simulink model "pid_controller"  (R2021b)
settings: Solver=VariableStepAuto  StartTime=0.0  StopTime=10.0  RelTol=1e-3
values from neighbouring files (symbols this model uses):
  Kd = 0.5    [init.m]
  Ki = 1    [init.m]
  Kp = 0.001    [init.m]    (also in init.mat = 1)
settings Model: Creator=lordx  LastModifiedBy=lordx

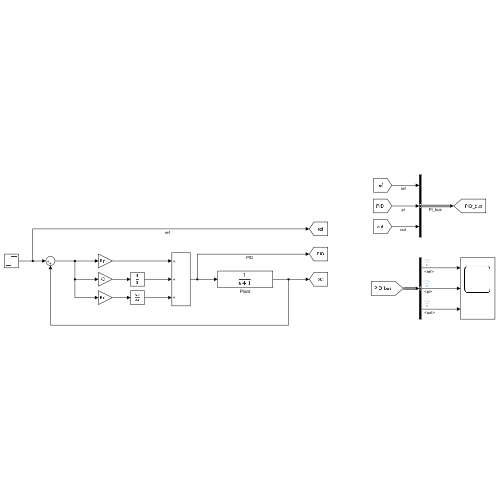
[thumbnail: Simulink's stored preview of the top-level diagram]
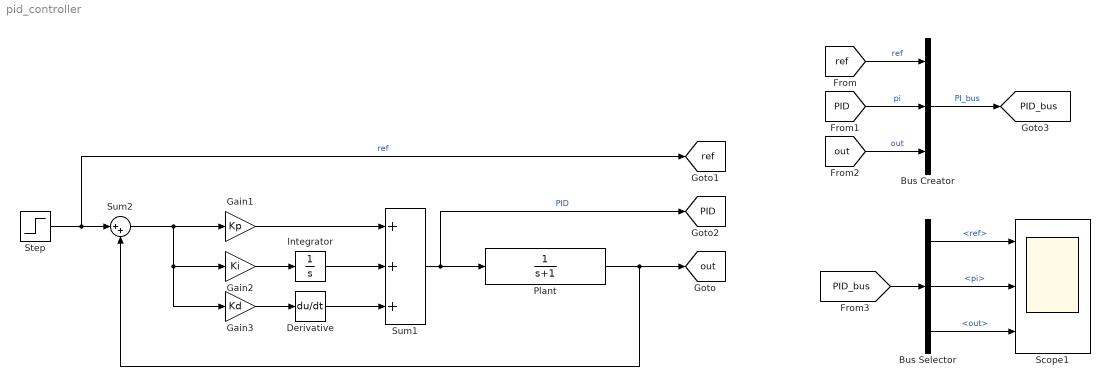
== system pid_controller ==
  Bus Selector : BusSelector  OutputSignals=ref,pi,out
  Bus Creator : BusCreator  Inputs=3
  Derivative : Derivative
  Gain1 : Gain  Gain=Kp
  Gain2 : Gain  Gain=Ki
  Gain3 : Gain  Gain=Kd
  Integrator : Integrator
  Plant : TransferFcn  Denominator=[1 1]
  Scope1 : Scope  NumInputPorts=3
  Step : Step  Time=0  SampleTime=0
  Sum1 : Sum  Inputs=+++
  Sum2 : Sum  Inputs=|++
  tag scope: PID=global, PID_bus=global, out=global, ref=global
  wires:
  Bus Creator/1 -> [PID_bus]  "PI_bus"
  Step/1 -> [ref], Sum2/1  "ref"
  Gain3/1 -> Derivative/1
  Derivative/1 -> Sum1/3
  [PID] -> Bus Creator/2  "pi"
  Sum1/1 -> [PID], Plant/1  "PID"
  [PID_bus] -> Bus Selector/1
  Bus Selector/2 -> Scope1/2  "<pi>"
  Bus Selector/1 -> Scope1/1  "<ref>"
  Integrator/1 -> Sum1/2
  [out] -> Bus Creator/3  "out"
  Gain1/1 -> Sum1/1
  Plant/1 -> [out], Sum2/2
  Sum2/1 -> Gain3/1, Gain2/1, Gain1/1
  [ref] -> Bus Creator/1  "ref"
  Gain2/1 -> Integrator/1
  Bus Selector/3 -> Scope1/3  "<out>"
